simulink model "ADAS_Controller_SIL_Model"  (R2026a)
settings: Solver=FixedStepDiscrete  FixedStep=0.1
settings Model: Creator=mushu  LastModifiedBy=mushu

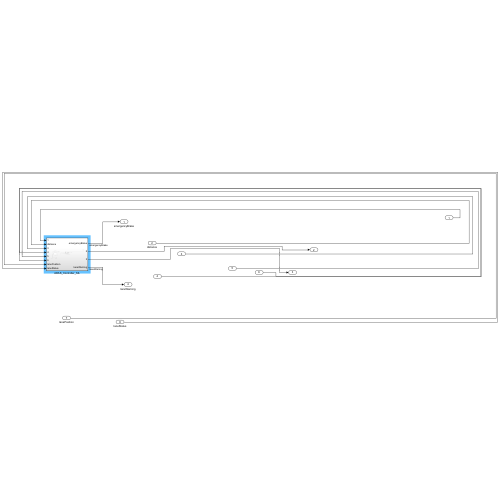
[thumbnail: Simulink's stored preview of the top-level diagram]
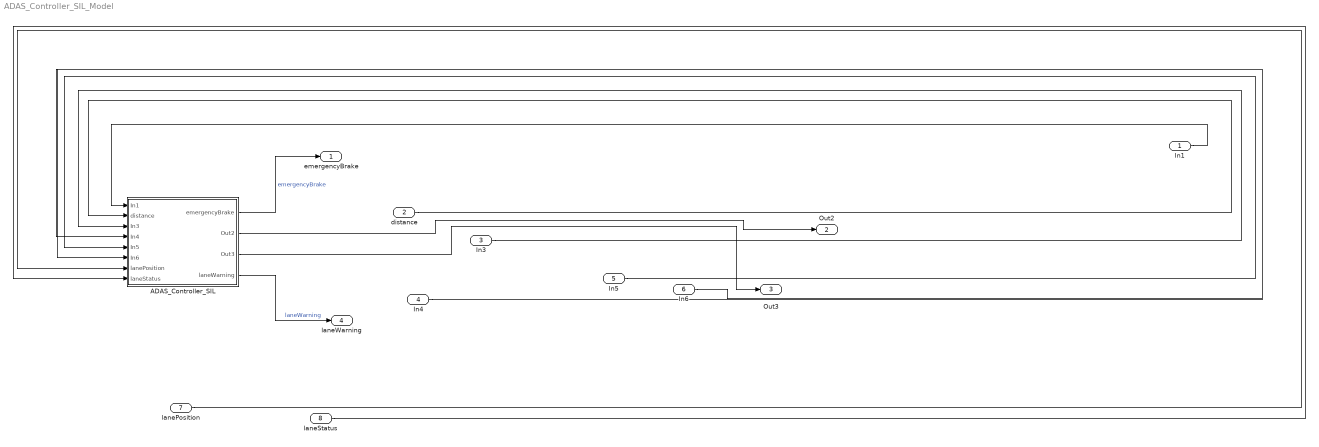
== system ADAS_Controller_SIL_Model ==
  In1 : Inport  OutDataTypeStr=uint8  PortDimensions=1  SampleTime=0.1
  distance : Inport  Port=2  OutDataTypeStr=double  PortDimensions=1  SampleTime=0.1
  In3 : Inport  Port=3  OutDataTypeStr=boolean  PortDimensions=1  SampleTime=0.1
  In4 : Inport  Port=4  OutDataTypeStr=boolean  PortDimensions=1  SampleTime=0.1
  In5 : Inport  Port=5  OutDataTypeStr=double  PortDimensions=1  SampleTime=0.1
  In6 : Inport  Port=6  OutDataTypeStr=double  PortDimensions=1  SampleTime=0.1
  lanePosition : Inport  Port=7  OutDataTypeStr=double  PortDimensions=[1 1]  SampleTime=0.1
  laneStatus : Inport  Port=8  OutDataTypeStr=double  PortDimensions=[1 1]  SampleTime=0.1
  ADAS_Controller_SIL : Subsystem
  emergencyBrake : Outport  OutDataTypeStr=double  PortDimensions=1  SampleTime=[0.10000000000000001,0]
  Out2 : Outport  Port=2  OutDataTypeStr=double  PortDimensions=1  SampleTime=[0.10000000000000001,0]
  Out3 : Outport  Port=3  OutDataTypeStr=double  PortDimensions=1  SampleTime=[0.10000000000000001,0]
  laneWarning : Outport  Port=4  OutDataTypeStr=double  PortDimensions=1  SampleTime=[0.10000000000000001,0]
  wires:
  In6/1 -> ADAS_Controller_SIL/6(In6)
  In5/1 -> ADAS_Controller_SIL/5(In5)
  distance/1 -> ADAS_Controller_SIL/2(distance)
  In4/1 -> ADAS_Controller_SIL/4(In4)
  laneStatus/1 -> ADAS_Controller_SIL/8(laneStatus)
  In1/1 -> ADAS_Controller_SIL/1(In1)
  ADAS_Controller_SIL/3(Out3) -> Out3/1
  In3/1 -> ADAS_Controller_SIL/3(In3)
  lanePosition/1 -> ADAS_Controller_SIL/7(lanePosition)
  ADAS_Controller_SIL/2(Out2) -> Out2/1
  ADAS_Controller_SIL/4(laneWarning) -> laneWarning/1  "laneWarning"
  ADAS_Controller_SIL/1(emergencyBrake) -> emergencyBrake/1  "emergencyBrake"

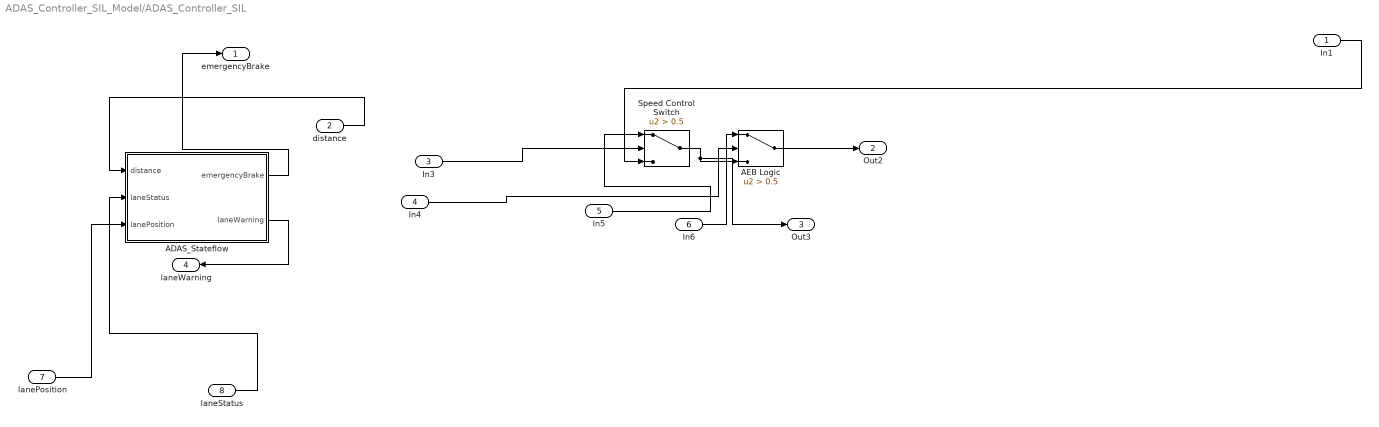
== system ADAS_Controller_SIL_Model/ADAS_Controller_SIL ==
  In1 : Inport
  distance : Inport  Port=2
  In3 : Inport  Port=3  SampleTime=0.1
  In4 : Inport  Port=4  SampleTime=0.1
  In5 : Inport  Port=5  SampleTime=0.1
  In6 : Inport  Port=6  SampleTime=0.1
  lanePosition : Inport  Port=7
  laneStatus : Inport  Port=8
  ADAS_Stateflow : Stateflow chart  TreatAsAtomicUnit=on
  AEB Logic : Switch  Criteria=u2 > Threshold  Threshold=0.5  SaturateOnIntegerOverflow=off  InputSameDT=off
  Speed Control Switch : Switch  Criteria=u2 > Threshold  Threshold=0.5  SaturateOnIntegerOverflow=off  InputSameDT=off
  emergencyBrake : Outport
  Out2 : Outport  Port=2
  Out3 : Outport  Port=3
  laneWarning : Outport  Port=4
  wires:
  ADAS_Stateflow/1(emergencyBrake) -> emergencyBrake/1
  distance/1 -> ADAS_Stateflow/1(distance)
  ADAS_Stateflow/2(laneWarning) -> laneWarning/1
  In4/1 -> AEB Logic/2
  lanePosition/1 -> ADAS_Stateflow/3(lanePosition)
  In6/1 -> AEB Logic/1
  laneStatus/1 -> ADAS_Stateflow/2(laneStatus)
  AEB Logic/1 -> Out2/1
  In5/1 -> Speed Control Switch/1
  In1/1 -> Speed Control Switch/3
  Speed Control Switch/1 -> AEB Logic/3, Out3/1
  In3/1 -> Speed Control Switch/2

== stateflow chart ADAS_Controller_SIL_Model/ADAS_Controller_SIL/ADAS_Stateflow ==
  state Normal
    entry:
    emergencyBrake = 0;
    laneWarning = 0;
  state Warning
    entry:
    emergencyBrake = 0;
    laneWarning = 0;
    during:
    laneWarning = double((laneStatus == 1) || (lanePosition ~= 0));
  state Emergency
    entry:
    emergencyBrake = 1;
    laneWarning = 0;
    during:
    laneWarning = laneStatus;
  (default) -> Normal
  Emergency -> Warning : [distance >= 10]
  Normal -> Warning : [distance < 20]
  Warning -> Normal [order 2] : [distance >= 20]
  Warning -> Emergency [order 1] : [distance < 10]
  data: distance input double =input; emergencyBrake output double; laneWarning output double; laneStatus input; lanePosition input
